simulink model "E5"  (Simulink 10.0)
settings: Solver=ode45  StartTime=0.0  StopTime=10^11  RelTol=1e-3  EnableMultiTasking=on
settings Model: Creator=UX31  LastModifiedBy=unknown
settings DataIOCC: LimitDataPoints=on
settings DebuggingCC: UnderspecifiedInitializationDetection=Simplified  MergeDetectMultiDrivingBlocksExec=error
settings GRTTargetCC: GeneratePreprocessorConditionals=Disable all  CombineOutputUpdateFcns=on  GRTInterface=off
settings ConfigComp: CovExternalEMLEnable=off  CovSFcnEnable=off

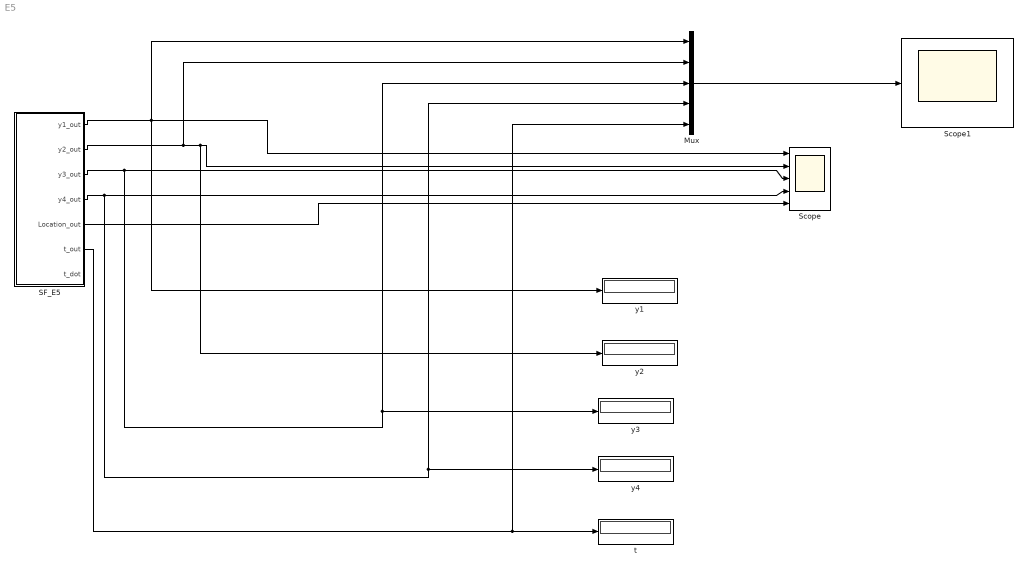
== system E5 ==
  Mux : Mux  Inputs=5
  SF_E5 : Stateflow chart  TreatAsAtomicUnit=on
  Scope : Scope  NumInputPorts=5
  Scope1 : Scope
  t : Display
  y{1..4} (4 alike) : Display
  wires:
  SF_E5/1(y1_out) -> Mux/1, y1/1, Scope/1
  SF_E5/2(y2_out) -> Mux/2, y2/1, Scope/2
  SF_E5/3(y3_out) -> Mux/3, y3/1, Scope/3
  SF_E5/4(y4_out) -> Mux/4, y4/1, Scope/4
  SF_E5/5(Location_out) -> Scope/5
  SF_E5/6(t_out) -> Mux/5, t/1
  Mux/1 -> Scope1/1

== stateflow chart SF_E5 ==
  settings: updateMethod=CONTINUOUS
  state E5
    du:
    y1_dot=-7.89*10^-10*y1-1.1*10^7*y1*y3;
    y2_dot=7.89*10^-10*y1-1.13*10^9*y2*y3;
    y3_dot=7.89*10^-10*y1-1.1*10^7*y1*y3-1.13*10^9*y2*y3+1.13*10^3*y4;
    y4_dot=1.1*10^7*y1*y3-1.13*10^3*y4;
    y1_out=y1;
    y2_out=y2;
    y3_out=y3;
    y4_out=y4;
    Location_out =1;
  state running_time
    du:
    t_dot=1;
    t_out=t;
    Location_out =1;
  (default) -> E5 [order 1] : {y1=1.76*10^-3; y2 = 0; y3=0; y4 = 0}
  (default) -> running_time [order 2]
  data: y1 local double; y1_out output double; y2 local double; y2_out output double; y3 local double; y3_out output double; y4 local double; y4_out output double; Location_out output double; t local double; t_out output double; t_dot output double; C constant double; A constant double; B constant double; M constant double
  data y1 settings: updateMethod=SF_CONTINUOUS_TIME_DATA
  data y2 settings: updateMethod=SF_CONTINUOUS_TIME_DATA
  data y3 settings: updateMethod=SF_CONTINUOUS_TIME_DATA
  data y4 settings: updateMethod=SF_CONTINUOUS_TIME_DATA
